simulink model "TST_CoVM_TrqDesCoord"  (R2016b)
settings: Solver=FixedStepDiscrete  StartTime=0.0  StopTime=simTime  FixedStep=sampleTime  RelTol=1e-3
values from neighbouring files (symbols this model uses):
  testCase = 1    [initTST_CoVM_TrqDesCoord_001.m]
libraries: simulink x3, UnitTest_Lib x1
settings Model: Creator=zhengjinyan  LastModifiedBy=zhengjinyan
settings DebuggingCC: SignalRangeChecking=error

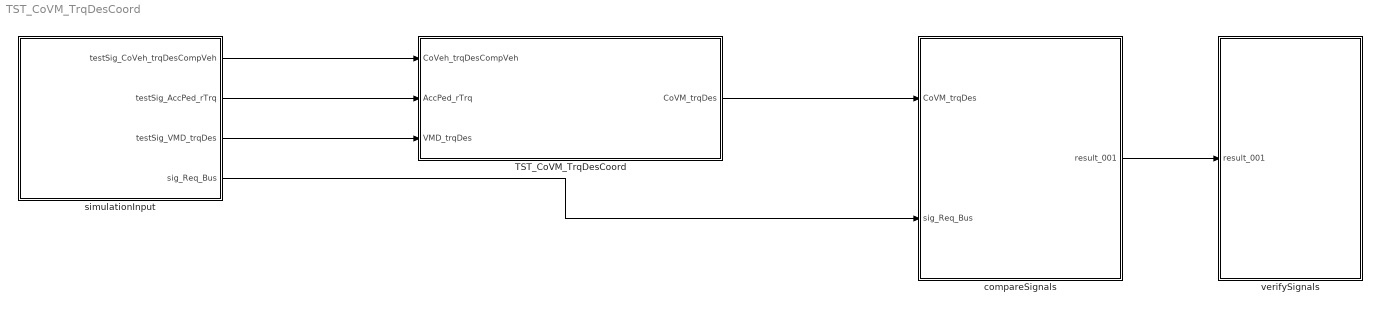
== system TST_CoVM_TrqDesCoord ==
  TST_CoVM_TrqDesCoord : Subsystem
  compareSignals : Subsystem
  simulationInput : Subsystem
  verifySignals : Subsystem
  wires:
  simulationInput/1(testSig_CoVeh_trqDesCompVeh) -> TST_CoVM_TrqDesCoord/1(CoVeh_trqDesCompVeh)
  simulationInput/2(testSig_AccPed_rTrq) -> TST_CoVM_TrqDesCoord/2(AccPed_rTrq)
  simulationInput/3(testSig_VMD_trqDes) -> TST_CoVM_TrqDesCoord/3(VMD_trqDes)
  TST_CoVM_TrqDesCoord/1(CoVM_trqDes) -> compareSignals/1(CoVM_trqDes)
  simulationInput/4(sig_Req_Bus) -> compareSignals/2(sig_Req_Bus)
  compareSignals/1(result_001) -> verifySignals/1(result_001)

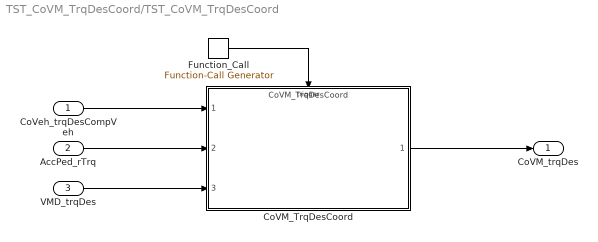
== system TST_CoVM_TrqDesCoord/TST_CoVM_TrqDesCoord ==
  CoVeh_trqDesCompVeh : Inport
  AccPed_rTrq : Inport  Port=2
  VMD_trqDes : Inport  Port=3
  CoVM_TrqDesCoord : ModelReference  ModelNameDialog=CoVM_TrqDesCoord  SimulationMode=Normal  ModelReferenceVersion=1.5  TriggerPortName=function  TriggerPortTriggerType=function-call  TriggerPortStatesWhenEnabling=held
  Function_Call : simulink/Ports & Subsystems/Function-Call Generator  sample_time=sampleTime  numberOfIterations=1
  CoVM_trqDes : Outport
  wires:
  Function_Call/1 -> CoVM_TrqDesCoord/Trigger
  CoVeh_trqDesCompVeh/1 -> CoVM_TrqDesCoord/1
  AccPed_rTrq/1 -> CoVM_TrqDesCoord/2
  VMD_trqDes/1 -> CoVM_TrqDesCoord/3
  CoVM_TrqDesCoord/1 -> CoVM_trqDes/1

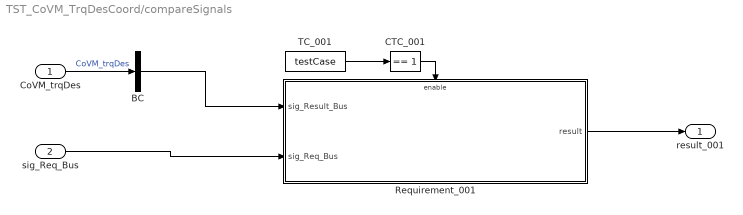
== system TST_CoVM_TrqDesCoord/compareSignals ==
  CoVM_trqDes : Inport
  sig_Req_Bus : Inport  Port=2
  BC : BusCreator  Inputs=1
  CTC_001 : simulink/Logic and Bit Operations/Compare To Constant  relop===  const=1  OutDataTypeStr=boolean
  Requirement_001 : Subsystem
  TC_001 : Constant  Value=testCase
  result_001 : Outport
  wires:
  CoVM_trqDes/1 -> BC/1  "CoVM_trqDes"
  TC_001/1 -> CTC_001/1
  CTC_001/1 -> Requirement_001/Enable
  sig_Req_Bus/1 -> Requirement_001/2(sig_Req_Bus)
  BC/1 -> Requirement_001/1(sig_Result_Bus)
  Requirement_001/1(result) -> result_001/1

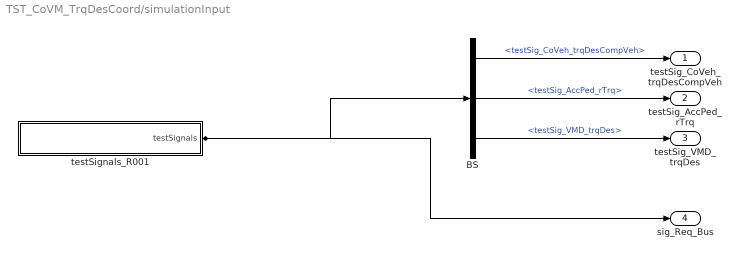
== system TST_CoVM_TrqDesCoord/simulationInput ==
  BS : BusSelector  OutputSignals=testSig_CoVeh_trqDesCompVeh,testSig_AccPed_rTrq,testSig_VMD_trqDes
  testSignals_R001 : Subsystem
  testSig_CoVeh_trqDesCompVeh : Outport
  testSig_AccPed_rTrq : Outport  Port=2
  testSig_VMD_trqDes : Outport  Port=3
  sig_Req_Bus : Outport  Port=4
  wires:
  BS/1 -> testSig_CoVeh_trqDesCompVeh/1  "<testSig_CoVeh_trqDesCompVeh>"
  BS/2 -> testSig_AccPed_rTrq/1  "<testSig_AccPed_rTrq>"
  BS/3 -> testSig_VMD_trqDes/1  "<testSig_VMD_trqDes>"
  testSignals_R001/1(testSignals) -> BS/1, sig_Req_Bus/1

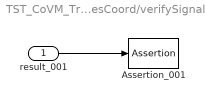
== system TST_CoVM_TrqDesCoord/verifySignals ==
  result_001 : Inport
  Assertion_001 : Assertion  Enabled=off
  wires:
  result_001/1 -> Assertion_001/1

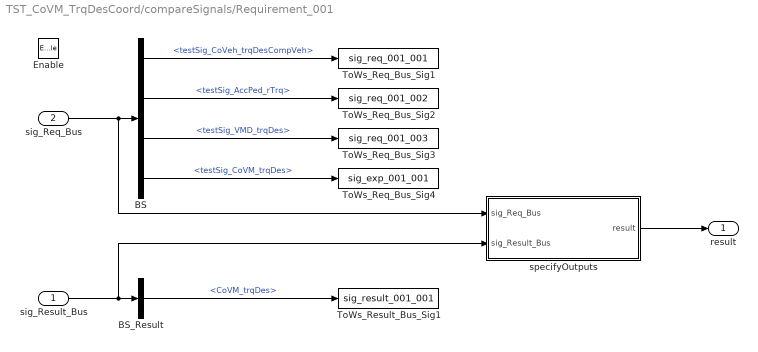
== system TST_CoVM_TrqDesCoord/compareSignals/Requirement_001 ==
  sig_Result_Bus : Inport
  sig_Req_Bus : Inport  Port=2
  Enable : EnablePort
  BS : BusSelector  OutputSignals=testSig_CoVeh_trqDesCompVeh,testSig_AccPed_rTrq,testSig_VMD_trqDes,testSig_CoVM_trqDes
  BS_Result : BusSelector  OutputSignals=CoVM_trqDes
  ToWs_Req_Bus_Sig1 : ToWorkspace  VariableName=sig_req_001_001  SaveFormat=Structure With Time
  ToWs_Req_Bus_Sig2 : ToWorkspace  VariableName=sig_req_001_002  SaveFormat=Structure With Time
  ToWs_Req_Bus_Sig3 : ToWorkspace  VariableName=sig_req_001_003  SaveFormat=Structure With Time
  ToWs_Req_Bus_Sig4 : ToWorkspace  VariableName=sig_exp_001_001  SaveFormat=Structure With Time
  ToWs_Result_Bus_Sig1 : ToWorkspace  VariableName=sig_result_001_001  SaveFormat=Structure With Time
  specifyOutputs : Subsystem
  result : Outport
  wires:
  sig_Req_Bus/1 -> BS/1, specifyOutputs/1(sig_Req_Bus)
  BS/1 -> ToWs_Req_Bus_Sig1/1  "<testSig_CoVeh_trqDesCompVeh>"
  BS/2 -> ToWs_Req_Bus_Sig2/1  "<testSig_AccPed_rTrq>"
  BS/3 -> ToWs_Req_Bus_Sig3/1  "<testSig_VMD_trqDes>"
  BS/4 -> ToWs_Req_Bus_Sig4/1  "<testSig_CoVM_trqDes>"
  sig_Result_Bus/1 -> BS_Result/1, specifyOutputs/2(sig_Result_Bus)
  BS_Result/1 -> ToWs_Result_Bus_Sig1/1  "<CoVM_trqDes>"
  specifyOutputs/1(result) -> result/1

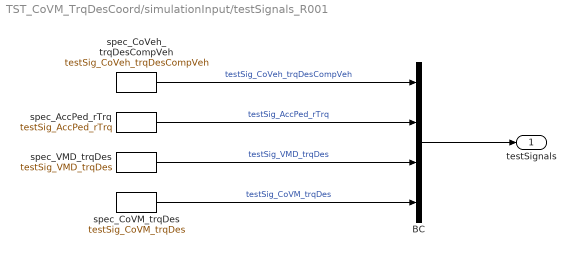
== system TST_CoVM_TrqDesCoord/simulationInput/testSignals_R001 ==
  BC : BusCreator  Inputs=4
  spec_AccPed_rTrq : FromWorkspace  VariableName=testSig_AccPed_rTrq  Interpolate=off  OutputAfterFinalValue=Holding final value
  spec_CoVM_trqDes : FromWorkspace  VariableName=testSig_CoVM_trqDes  Interpolate=off  OutputAfterFinalValue=Holding final value
  spec_CoVeh_trqDesCompVeh : FromWorkspace  VariableName=testSig_CoVeh_trqDesCompVeh  Interpolate=off  OutputAfterFinalValue=Holding final value
  spec_VMD_trqDes : FromWorkspace  VariableName=testSig_VMD_trqDes  Interpolate=off  OutputAfterFinalValue=Holding final value
  testSignals : Outport
  wires:
  BC/1 -> testSignals/1
  spec_CoVeh_trqDesCompVeh/1 -> BC/1  "testSig_CoVeh_trqDesCompVeh"
  spec_AccPed_rTrq/1 -> BC/2  "testSig_AccPed_rTrq"
  spec_VMD_trqDes/1 -> BC/3  "testSig_VMD_trqDes"
  spec_CoVM_trqDes/1 -> BC/4  "testSig_CoVM_trqDes"

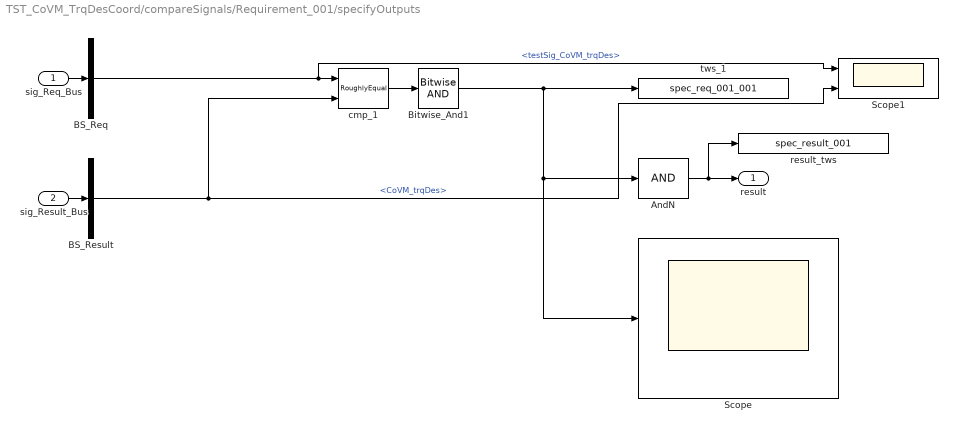
== system TST_CoVM_TrqDesCoord/compareSignals/Requirement_001/specifyOutputs ==
  sig_Req_Bus : Inport
  sig_Result_Bus : Inport  Port=2
  AndN : Logic  Inputs=1
  BS_Req : BusSelector  OutputSignals=testSig_CoVM_trqDes
  BS_Result : BusSelector  OutputSignals=CoVM_trqDes
  Bitwise_And1 : simulink/Logic and Bit Operations/Bitwise Operator  logicop=AND  UseBitMask=off  BitMask=bin2dec('11011001')  BitMaskRealWorld=Stored Integer
  Scope : Scope
  Scope1 : Scope  NumInputPorts=2
  cmp_1 : UnitTest_Lib/RoughlyEqual  slope=1
  result_tws : ToWorkspace  VariableName=spec_result_001
  tws_1 : ToWorkspace  VariableName=spec_req_001_001
  result : Outport
  wires:
  sig_Req_Bus/1 -> BS_Req/1
  sig_Result_Bus/1 -> BS_Result/1
  AndN/1 -> result/1, result_tws/1
  BS_Req/1 -> cmp_1/1, Scope1/1  "<testSig_CoVM_trqDes>"
  BS_Result/1 -> cmp_1/2, Scope1/2  "<CoVM_trqDes>"
  cmp_1/1 -> Bitwise_And1/1
  Bitwise_And1/1 -> AndN/1, Scope/1, tws_1/1
